simulink model "svpwm"  (R2024b)
settings: Solver=FixedStepAuto  StartTime=0.0  StopTime=0.02  FixedStep=1e-6  RelTol=1e-3
libraries: spsIGBTDiodeLib x6, simulink x5, spsDCVoltageSourceLib x1, spsThreePhaseSeriesRLCLoadLib x1, spsThreePhaseVIMeasurementLib x1, sps_lib x1
settings Model: Creator=killa  LastModifiedBy=killa

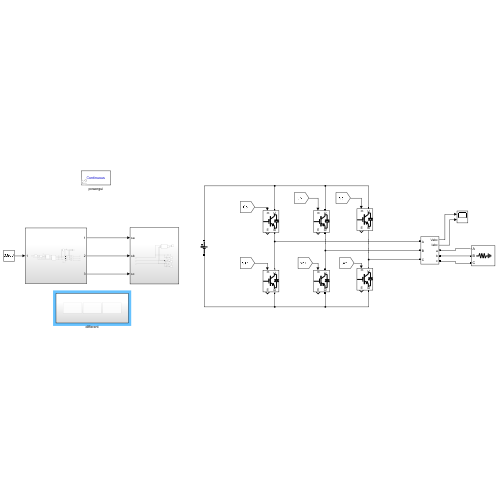
[thumbnail: Simulink's stored preview of the top-level diagram]
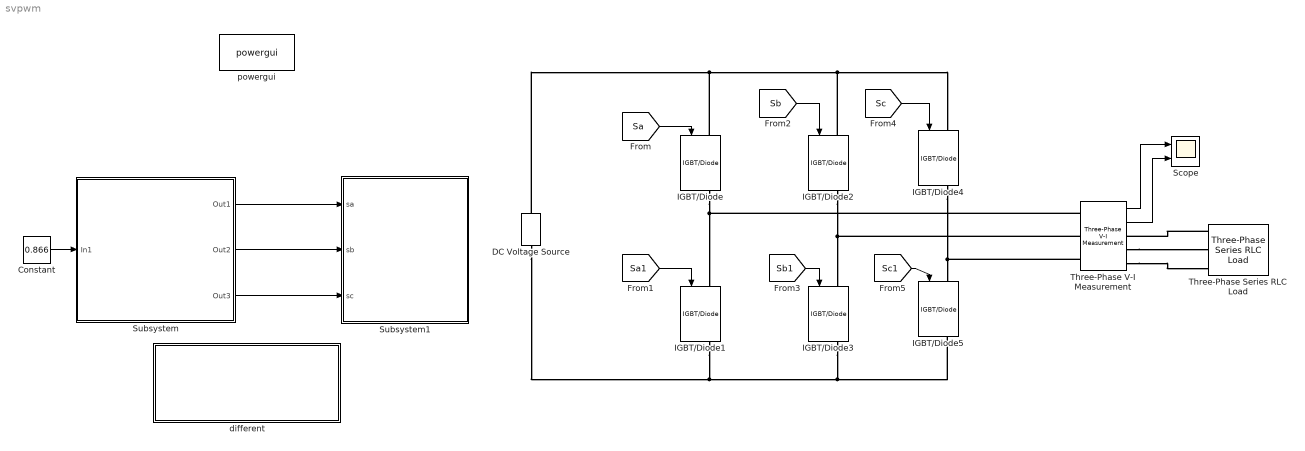
== system svpwm ==
  Constant : Constant  Value=0.866
  DC Voltage Source : spsDCVoltageSourceLib/DC Voltage Source  Amplitude=600  Measurements=None
  IGBT/Diode{,1..5} (6 alike) : spsIGBTDiodeLib/IGBT//Diode  Ron=1e-3  Rs=1e5  Cs=inf  Measurements=on
  Scope : Scope  NumInputPorts=2
  Subsystem : Subsystem
  Subsystem1 : Subsystem
  Three-Phase Series RLC Load : spsThreePhaseSeriesRLCLoadLib/Three-Phase Series RLC Load  LConnTagsString=A|B|C  Configuration=Y (grounded)  NominalVoltage=415  Vabc=[1e3 1e3 1e3]  Vabcp=[1e3 1e3 1e3]  NominalFrequency=50  UnbalancedPower=off  ActivePower=10e3  InductivePower=0  CapacitivePower=0  Pabc=[10e3 9e3 11e3]  QLabc=[100 90 110]  QCabc=[100 90 110]  Pabcp=[10e3 9e3 11e3]  QLabcp=[100 90 110]  QCabcp=[100 90 110]  Measurements=Branch currents  LoadType=constant Z
  Three-Phase V-I Measurement : spsThreePhaseVIMeasurementLib/Three-Phase V-I Measurement  VoltageMeasurement=phase-to-ground  SetLabelV=off  LabelV=Vabc  Vpu=off  VpuLL=off  CurrentMeasurement=yes  SetLabelI=off  LabelI=Iabc  Ipu=off  Pbase=100e6  Vbase=500e3  OutputType=Complex  PhasorSimulation=off  PSBequivalent=0
  different : Subsystem
  powergui : sps_lib/powergui  Priority=1  SimulationMode=Continuous  SampleTime=1e-6  frequency=60  Iterations=50  frequencyindice=0  Pbase=100e6  ErrMax=1e-4  UnitsV=kV  UnitsW=MW  buscounter=0  FunctionMessages=off  echomessages=off  EnableUseOfTLC=off  CurrentSourceSwitches=off  DisableSnubberDevices=off  DisableRonSwitches=off  DisableVfSwitches=off  DisplayEquations=off  AutomaticDiscreteSolvers=off  SolverType=Tustin/Backward Euler (TBE)  Interpol=off  ExternalGateDelay=off  methode=off  Ts=100  x0status=blocks  SPID=on  SwTol=0  HookPort=off  NonlinearTolerance=1e-4  nMaxIteration=100  ContinueOnMaxIteration=off  RestoreLinks=warning  ResistiveCurrentMeasurement=off  Frange=[0:2:500]  Ylog=off  Xlog=on  ShowGrid=off  save=off  variable=ZData  structure=0  ZoomFFT=off  StartTime=0.0  cycles=1  DisplayStyle=1  fundamental=60  FreqAxis=off  MaxFrequency=1000  frequencyindicesteady=1  RmsSteady=1  display=off
  wires:
  [Sa1] -> IGBT/Diode1/1
  [Sa] -> IGBT/Diode/1
  [Sb] -> IGBT/Diode2/1
  [Sb1] -> IGBT/Diode3/1
  [Sc] -> IGBT/Diode4/1
  [Sc1] -> IGBT/Diode5/1
  Three-Phase V-I Measurement/1 -> Scope/1
  Three-Phase V-I Measurement/2 -> Scope/2
  Constant/1 -> Subsystem/1(In1)
  Subsystem/1(Out1) -> Subsystem1/1(sa)
  Subsystem/2(Out2) -> Subsystem1/2(sb)
  Subsystem/3(Out3) -> Subsystem1/3(sc)
  connections:
  IGBT/Diode/LConn1 -- DC Voltage Source/RConn1 -- IGBT/Diode4/LConn1 -- IGBT/Diode2/LConn1
  IGBT/Diode/RConn1 -- Three-Phase V-I Measurement/LConn1 -- IGBT/Diode1/LConn1
  IGBT/Diode2/RConn1 -- Three-Phase V-I Measurement/LConn2 -- IGBT/Diode3/LConn1
  IGBT/Diode4/RConn1 -- Three-Phase V-I Measurement/LConn3 -- IGBT/Diode5/LConn1
  IGBT/Diode1/RConn1 -- DC Voltage Source/LConn1 -- IGBT/Diode3/RConn1 -- IGBT/Diode5/RConn1
  Three-Phase Series RLC Load/LConn1 -- Three-Phase V-I Measurement/RConn1
  Three-Phase V-I Measurement/RConn2 -- Three-Phase Series RLC Load/LConn2
  Three-Phase V-I Measurement/RConn3 -- Three-Phase Series RLC Load/LConn3

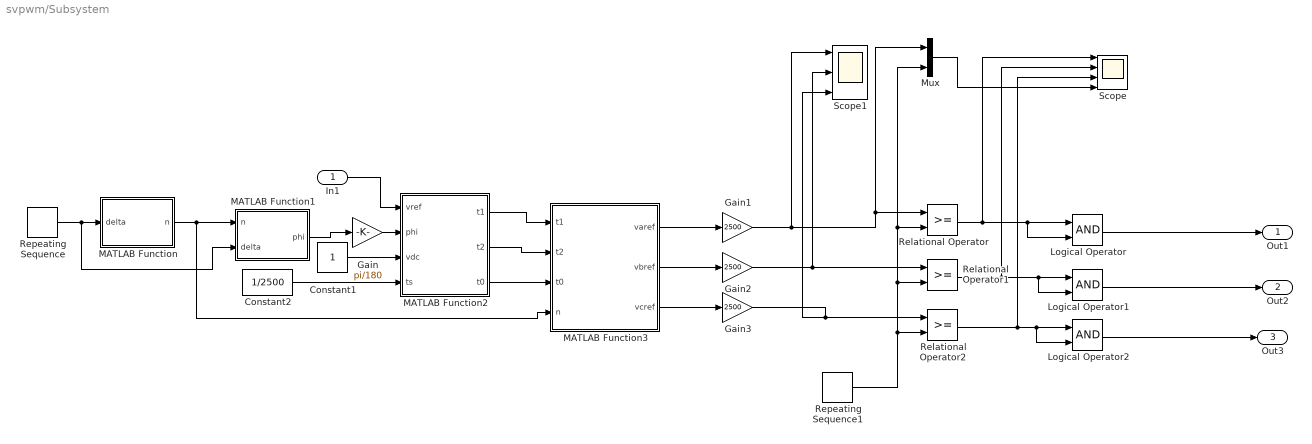
== system svpwm/Subsystem ==
  In1 : Inport
  Constant1 : Constant
  Constant2 : Constant  Value=1/2500
  Gain : Gain  Gain=pi/180
  Gain1 : Gain  Gain=2500
  Gain2 : Gain  Gain=2500
  Gain3 : Gain  Gain=2500
  Logical Operator : Logic  AllPortsSameDT=off  OutDataTypeStr=boolean
  Logical Operator1 : Logic  AllPortsSameDT=off  OutDataTypeStr=boolean
  Logical Operator2 : Logic  AllPortsSameDT=off  OutDataTypeStr=boolean
  MATLAB Function : MATLAB Function  TreatAsAtomicUnit=on
  MATLAB Function1 : MATLAB Function  TreatAsAtomicUnit=on
  MATLAB Function2 : MATLAB Function  TreatAsAtomicUnit=on
  MATLAB Function3 : MATLAB Function  TreatAsAtomicUnit=on
  Mux : Mux  Inputs=2
  Relational Operator : RelationalOperator  OutDataTypeStr=boolean  RndMeth=Simplest  InputSameDT=off
  Relational Operator1 : RelationalOperator  OutDataTypeStr=boolean  RndMeth=Simplest  InputSameDT=off
  Relational Operator2 : RelationalOperator  OutDataTypeStr=boolean  RndMeth=Simplest  InputSameDT=off
  Repeating Sequence : simulink/Sources/Repeating Sequence  rep_seq_t=[0 0.02]  rep_seq_y=[0 360]
  Repeating Sequence1 : simulink/Sources/Repeating Sequence  rep_seq_t=[0 0.5 1]/2500  rep_seq_y=[0 1 0]
  Scope : Scope  NumInputPorts=4
  Scope1 : Scope  NumInputPorts=3
  Out1 : Outport
  Out2 : Outport  Port=2
  Out3 : Outport  Port=3
  wires:
  Constant2/1 -> MATLAB Function2/4(ts)
  Repeating Sequence/1 -> MATLAB Function1/2(delta), MATLAB Function/1(delta)
  In1/1 -> MATLAB Function2/1(vref)
  Logical Operator/1 -> Out1/1
  MATLAB Function3/3(vcref) -> Gain3/1
  Logical Operator1/1 -> Out2/1
  Repeating Sequence1/1 -> Relational Operator2/2, Relational Operator1/2, Relational Operator/2, Mux/2
  MATLAB Function2/1(t1) -> MATLAB Function3/1(t1)
  Gain1/1 -> Scope1/1, Mux/1, Relational Operator/1
  Relational Operator/1 -> Scope/1, Logical Operator/2, Logical Operator/1
  Gain3/1 -> Relational Operator2/1, Scope1/3
  MATLAB Function2/3(t0) -> MATLAB Function3/3(t0)
  MATLAB Function3/1(varef) -> Gain1/1
  MATLAB Function2/2(t2) -> MATLAB Function3/2(t2)
  Relational Operator1/1 -> Scope/2, Logical Operator1/2, Logical Operator1/1
  Gain/1 -> MATLAB Function2/2(phi)
  MATLAB Function3/2(vbref) -> Gain2/1
  MATLAB Function1/1(phi) -> Gain/1
  MATLAB Function/1(n) -> MATLAB Function1/1(n), MATLAB Function3/4(n)
  Relational Operator2/1 -> Scope/3, Logical Operator2/2, Logical Operator2/1
  Gain2/1 -> Relational Operator1/1, Scope1/2
  Constant1/1 -> MATLAB Function2/3(vdc)
  Logical Operator2/1 -> Out3/1
  Mux/1 -> Scope/4

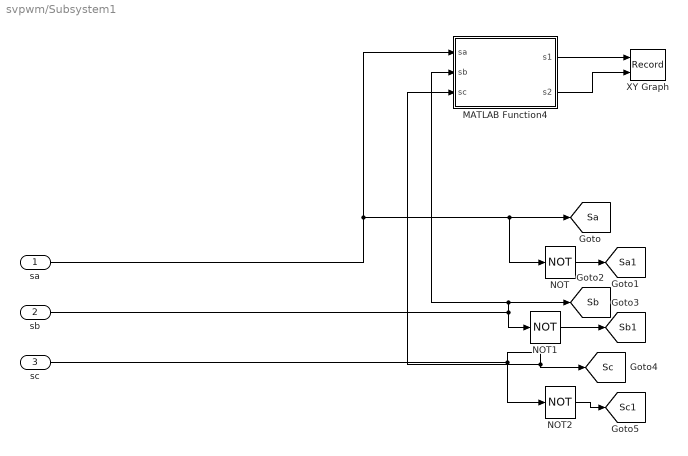
== system svpwm/Subsystem1 ==
  sa : Inport
  sb : Inport  Port=2
  sc : Inport  Port=3
  MATLAB Function4 : MATLAB Function  TreatAsAtomicUnit=on
  NOT : Logic  Operator=NOT  IconShape=distinctive  AllPortsSameDT=off  OutDataTypeStr=boolean
  NOT1 : Logic  Operator=NOT  IconShape=distinctive  AllPortsSameDT=off  OutDataTypeStr=boolean
  NOT2 : Logic  Operator=NOT  IconShape=distinctive  AllPortsSameDT=off  OutDataTypeStr=boolean
  XY Graph : Record  FileSettingsInternal="{\"entries\":[{\"content\":{\"excelSettings\":{\"content\":{},\"type\":\"Streamout.ExcelSettings\"}},\"type\":\"Streamout.FileSettingStorage\",\"uuid\":\"\"}],\"packageUris\":[\"http:\\/\\/schema.mathworks.com\\/mf0\\/streamout_blocks\\/R2020a\"],\"version\":\"1.0\"}"  Layout=[1 1]  SignalsInternal="{\"entries\":[{\"content\":{\"signals\":[{\"content\":{\"blockPath\":[],\"dimensions\":[1],\"domain\":\"\",\"lineColor\":\"#a2142f\",\"plots\":[ 1 ],\"port\":1,\"sid\":[\"\"],\"signalID\":1,\"signalName\":\"MATLAB Function4:1\"},\"type\":\"RecordBlkView.Signal\",\"uuid\":\"\"},{\"content\":{\"blockPath\":[],\"dimensions\":[1],\"domain\":\"\",\"lineColor\":\"#139fff\",\"plots\":[ 1 ],\"port\":2,\"sid\":[\"\"],\"signalID\":2,\"signalName\":\"MATLAB Function4:2\"},\"type\":\"RecordBlkView.Signal\",\"uuid\":\"\"}]},\"type\":\"RecordBlkView.InputSignals\",\"uuid\":\"\"}],\"packageUris\":[\"http:\\/\\/schema.mathworks.com\\/mf0\\/streamout_blocks\\/R2020a\"],\"version\":\"1.0\"}"  VisualizationBindings="{\"xyplotplugin\":{\"info\":[{\"series\":[{\"bindingParametersList\":[{\"parameter\":\"X-Axis\",\"signalID\":1,\"signalName\":\"MATLAB Function4:1\"},{\"parameter\":\"Y-Axis\",\"signalID\":2,\"signalName\":\"MATLAB Function4:2\"}],\"seriesID\":0}],\"subplotID\":1}]}}"  CompatibilityTag=XY
  tag scope: Sa1=global, Sa=global, Sb1=global, Sb=global, Sc1=global, Sc=global
  wires:
  MATLAB Function4/2(s2) -> XY Graph/2
  sa/1 -> MATLAB Function4/1(sa), NOT/1, [Sa]
  MATLAB Function4/1(s1) -> XY Graph/1
  sc/1 -> MATLAB Function4/3(sc), [Sc], NOT2/1
  sb/1 -> [Sb], MATLAB Function4/2(sb), NOT1/1
  NOT1/1 -> [Sb1]
  NOT2/1 -> [Sc1]
  NOT/1 -> [Sa1]

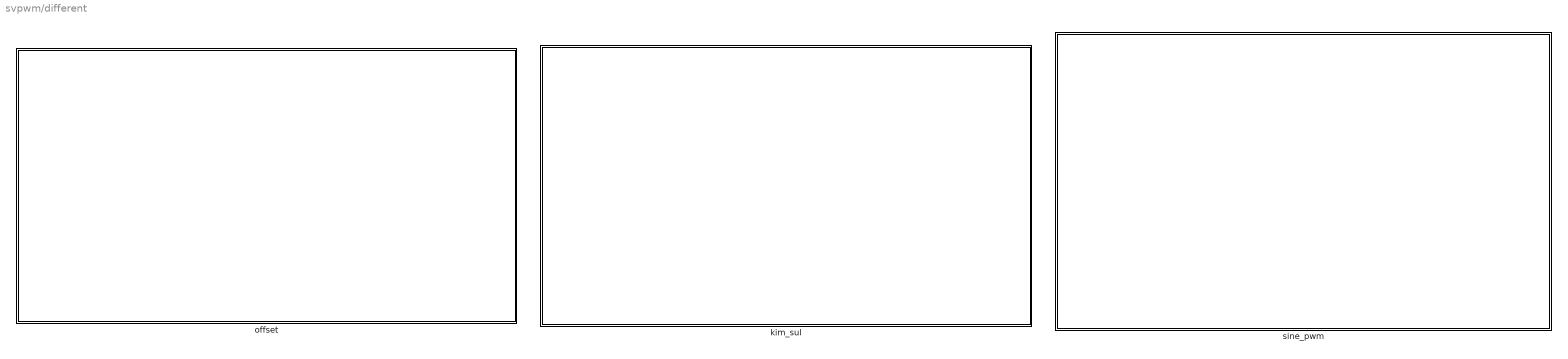
== system svpwm/different ==
  kim_sul : Subsystem
  offset : Subsystem
  sine_pwm : Subsystem

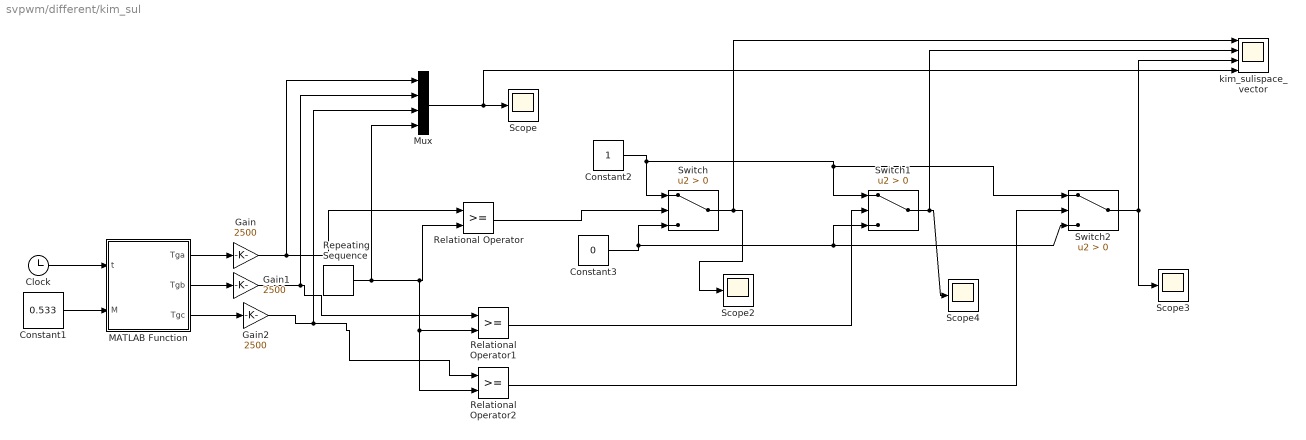
== system svpwm/different/kim_sul ==
  Clock : Clock
  Constant1 : Constant  Value=0.533
  Constant2 : Constant
  Constant3 : Constant  Value=0
  Gain : Gain  Gain=2500
  Gain1 : Gain  Gain=2500
  Gain2 : Gain  Gain=2500
  MATLAB Function : MATLAB Function  TreatAsAtomicUnit=on
  Mux : Mux
  Relational Operator : RelationalOperator  OutDataTypeStr=boolean  RndMeth=Simplest  InputSameDT=off
  Relational Operator1 : RelationalOperator  OutDataTypeStr=boolean  RndMeth=Simplest  InputSameDT=off
  Relational Operator2 : RelationalOperator  OutDataTypeStr=boolean  RndMeth=Simplest  InputSameDT=off
  Repeating Sequence : simulink/Sources/Repeating Sequence  rep_seq_t=[0 0.5 1]/2500  rep_seq_y=[0 1 0]
  Scope{,2..4} (4 alike) : Scope
  Switch : Switch  Criteria=u2 > Threshold  SaturateOnIntegerOverflow=off  InputSameDT=off
  Switch1 : Switch  Criteria=u2 > Threshold  SaturateOnIntegerOverflow=off  InputSameDT=off
  Switch2 : Switch  Criteria=u2 > Threshold  SaturateOnIntegerOverflow=off  InputSameDT=off
  kim_sulispace_vector : Scope  NumInputPorts=4
  wires:
  Repeating Sequence/1 -> Mux/4, Relational Operator2/2, Relational Operator1/2, Relational Operator/2
  MATLAB Function/1(Tga) -> Gain/1
  MATLAB Function/2(Tgb) -> Gain1/1
  MATLAB Function/3(Tgc) -> Gain2/1
  Constant1/1 -> MATLAB Function/2(M)
  Clock/1 -> MATLAB Function/1(t)
  Gain/1 -> Mux/1, Relational Operator/1
  Gain1/1 -> Mux/2, Relational Operator1/1
  Gain2/1 -> Mux/3, Relational Operator2/1
  Relational Operator2/1 -> Switch2/2
  Switch/1 -> kim_sulispace_vector/1, Scope2/1
  Constant3/1 -> Switch2/3, Switch1/3, Switch/3
  Constant2/1 -> Switch2/1, Switch1/1, Switch/1
  Relational Operator1/1 -> Switch1/2
  Switch1/1 -> kim_sulispace_vector/2, Scope4/1
  Relational Operator/1 -> Switch/2
  Switch2/1 -> kim_sulispace_vector/3, Scope3/1
  Mux/1 -> kim_sulispace_vector/4, Scope/1

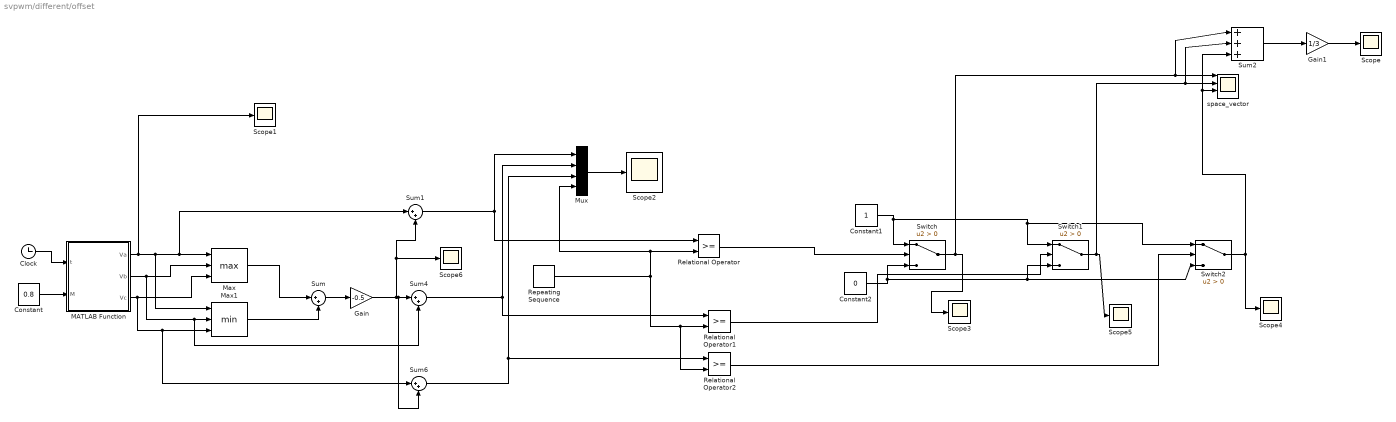
== system svpwm/different/offset ==
  Clock : Clock
  Constant : Constant  Value=0.8
  Constant1 : Constant
  Constant2 : Constant  Value=0
  Gain : Gain  Gain=-0.5
  Gain1 : Gain  Gain=1/3
  MATLAB Function : MATLAB Function  TreatAsAtomicUnit=on
  Max : MinMax  Function=max  Inputs=3
  Max1 : MinMax  Inputs=3
  Mux : Mux
  Relational Operator : RelationalOperator  OutDataTypeStr=boolean  RndMeth=Simplest  InputSameDT=off
  Relational Operator1 : RelationalOperator  OutDataTypeStr=boolean  RndMeth=Simplest  InputSameDT=off
  Relational Operator2 : RelationalOperator  OutDataTypeStr=boolean  RndMeth=Simplest  InputSameDT=off
  Repeating Sequence : simulink/Sources/Repeating Sequence  rep_seq_t=[0 0.5 1]/2500  rep_seq_y=[-1 1 -1]
  Scope{,1..6} (7 alike) : Scope
  Sum{,1,4,6} (4 alike) : Sum  Inputs=|++
  Sum2 : Sum  Inputs=|+++
  Switch : Switch  Criteria=u2 > Threshold  SaturateOnIntegerOverflow=off  InputSameDT=off
  Switch1 : Switch  Criteria=u2 > Threshold  SaturateOnIntegerOverflow=off  InputSameDT=off
  Switch2 : Switch  Criteria=u2 > Threshold  SaturateOnIntegerOverflow=off  InputSameDT=off
  space_vector : Scope  NumInputPorts=4
  wires:
  Sum/1 -> Gain/1
  Max/1 -> Sum/1
  Gain/1 -> Sum1/2, Scope6/1, Sum6/2, Sum4/1
  Max1/1 -> Sum/2
  Repeating Sequence/1 -> Relational Operator/2, Mux/4, Relational Operator2/2, Relational Operator1/2
  Clock/1 -> MATLAB Function/1(t)
  Sum1/1 -> Mux/1, Relational Operator/1
  Sum4/1 -> Mux/2, Relational Operator1/1
  Sum6/1 -> Mux/3, Relational Operator2/1
  Constant/1 -> MATLAB Function/2(M)
  MATLAB Function/1(Va) -> Scope1/1, Max1/1, Sum1/1, Max/1
  MATLAB Function/2(Vb) -> Sum4/2, Max1/2, Max/2
  MATLAB Function/3(Vc) -> Sum6/1, Max1/3, Max/3
  Switch1/1 -> Sum2/2, space_vector/2, Scope5/1
  Switch2/1 -> Sum2/3, space_vector/3, Scope4/1
  Switch/1 -> Sum2/1, space_vector/1, Scope3/1
  Constant2/1 -> Switch2/3, Switch1/3, Switch/3
  Relational Operator1/1 -> Switch1/2
  Constant1/1 -> Switch2/1, Switch1/1, Switch/1
  Relational Operator/1 -> Switch/2
  Relational Operator2/1 -> Switch2/2
  Sum2/1 -> Gain1/1
  Gain1/1 -> Scope/1
  Mux/1 -> Scope2/1

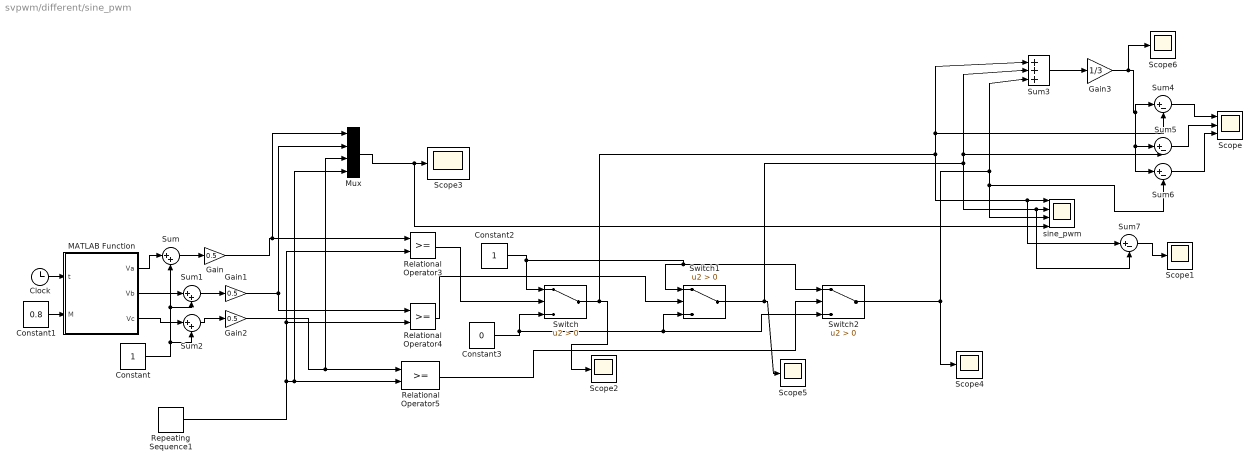
== system svpwm/different/sine_pwm ==
  Clock : Clock
  Constant : Constant
  Constant1 : Constant  Value=0.8
  Constant2 : Constant
  Constant3 : Constant  Value=0
  Gain : Gain  Gain=0.5
  Gain1 : Gain  Gain=0.5
  Gain2 : Gain  Gain=0.5
  Gain3 : Gain  Gain=1/3
  MATLAB Function : MATLAB Function  TreatAsAtomicUnit=on
  Mux : Mux
  Relational Operator3 : RelationalOperator  OutDataTypeStr=boolean  RndMeth=Simplest  InputSameDT=off
  Relational Operator4 : RelationalOperator  OutDataTypeStr=boolean  RndMeth=Simplest  InputSameDT=off
  Relational Operator5 : RelationalOperator  OutDataTypeStr=boolean  RndMeth=Simplest  InputSameDT=off
  Repeating Sequence1 : simulink/Sources/Repeating Sequence  rep_seq_t=[0 0.5 1]/2500  rep_seq_y=[0 1 0]
  Scope : Scope  NumInputPorts=3
  Scope{1..6} (6 alike) : Scope
  Sum : Sum  Inputs=|++
  Sum1 : Sum  Inputs=|++
  Sum2 : Sum  Inputs=|++
  Sum3 : Sum  Inputs=|+++
  Sum{4..7} (4 alike) : Sum  Inputs=|+-
  Switch : Switch  Criteria=u2 > Threshold  SaturateOnIntegerOverflow=off  InputSameDT=off
  Switch1 : Switch  Criteria=u2 > Threshold  SaturateOnIntegerOverflow=off  InputSameDT=off
  Switch2 : Switch  Criteria=u2 > Threshold  SaturateOnIntegerOverflow=off  InputSameDT=off
  sine_pwm : Scope  NumInputPorts=4
  wires:
  Repeating Sequence1/1 -> Relational Operator4/2, Relational Operator3/2, Mux/4, Relational Operator5/2
  Sum/1 -> Gain/1
  Sum1/1 -> Gain1/1
  Sum2/1 -> Gain2/1
  Constant/1 -> Sum2/2, Sum1/2, Sum/2
  Gain/1 -> Mux/1, Relational Operator3/1
  Gain1/1 -> Mux/2, Relational Operator4/1
  MATLAB Function/1(Va) -> Sum/1
  MATLAB Function/2(Vb) -> Sum1/1
  MATLAB Function/3(Vc) -> Sum2/1
  Clock/1 -> MATLAB Function/1(t)
  Constant1/1 -> MATLAB Function/2(M)
  Relational Operator4/1 -> Switch1/2
  Relational Operator3/1 -> Switch/2
  Relational Operator5/1 -> Switch2/2
  Sum6/1 -> Scope/3
  Switch1/1 -> Sum5/2, Sum3/2, Sum7/2, sine_pwm/2, Scope5/1
  Constant3/1 -> Switch2/3, Switch1/3, Switch/3
  Constant2/1 -> Switch2/1, Switch1/1, Switch/1
  Sum4/1 -> Scope/1
  Sum7/1 -> Scope1/1
  Switch2/1 -> Sum3/3, Sum6/2, sine_pwm/3, Scope4/1
  Gain3/1 -> Scope6/1, Sum6/1, Sum5/1, Sum4/1
  Sum3/1 -> Gain3/1
  Sum5/1 -> Scope/2
  Switch/1 -> Sum4/2, Sum3/1, Sum7/1, sine_pwm/1, Scope2/1
  Mux/1 -> sine_pwm/4, Scope3/1
  Gain2/1 -> Mux/3, Relational Operator5/1

== matlab function svpwm/Subsystem/MATLAB Function1 ==
  data: n input; delta input; phi output
function phi = phi(n,delta)
phi=0;
if n==1 
    phi=delta;
end
if n==2 
    phi=delta-60;
end
if n==3 
    phi=delta-120;
end
if n==4 
    phi=delta-180;
end
if n==5 
    phi=delta-240;
end
if n==6 
    phi=delta-300;
end

end

== matlab function svpwm/Subsystem/MATLAB Function ==
  data: delta input; n output
function n = sector(delta)
n=0;
if delta>=0 && delta<=60
    n=1;
end
if delta>=60 && delta<=120
    n=2;
end
if delta>=120 && delta<=180
    n=3;
end
if delta>=180 && delta<=240
    n=4;
end
if delta>=240 && delta<=300
    n=5;
end
if delta>=300 && delta<=360
    n=6;
end
end

== matlab function svpwm/Subsystem/MATLAB Function2 ==
  data: vref input; phi input; t1 output; vdc input; ts input; t2 output; t0 output
function [t1,t2,t0] = timings(vref,phi,vdc,ts)
t1=ts*(vref/vdc)*sin((pi/3)-phi)/sin(pi/3);
t2=ts*(vref/vdc)*sin(phi)/sin(pi/3);
t0=ts-(t1+t2);
end

== matlab function svpwm/Subsystem/MATLAB Function3 ==
  data: t1 input; t2 input; t0 input; n input; varef output; vbref output; vcref output
function [varef,vbref,vcref] = vref(t1,t2,t0,n)
varef=0;vbref=0;vcref=0;
if n==1
    varef=t1+t2+t0/2;
    vbref=t2+t0/2;
    vcref=t0/2;
end
if n==2
    varef=t1+t0/2;
    vbref=t1+t2+t0/2;
    vcref=t0/2;
end
if n==3
    varef=t0/2;
    vbref=t1+t2+t0/2;
    vcref=t2+t0/2;
end
if n==4
    varef=t0/2;
    vbref=t1+t0/2;
    vcref=t1+t2+t0/2;
end
if n==5
    varef=t2+t0/2;
    vbref=t0/2;
    vcref=t1+t2+t0/2;
end
if n==6
    varef=t1+t2+t0/2;
    vbref=t0/2;
    vcref=t1+t0/2;
end
end

== matlab function svpwm/Subsystem1/MATLAB Function4 ==
  data: sa input; s1 output; sb input; sc input; s2 output
function [s1,s2] = space_vector(sa,sb,sc)
s1=sa*cos(0)+sb*cos(2*pi/3)+sc*cos(4*pi/3);
s2=sa*sin(0)+sb*sin(2*pi/3)+sc*sin(4*pi/3);
end

== matlab function svpwm/different/kim_sul/MATLAB Function ==
  data: t input; Tga output; M input; Tgb output; Tgc output
function [Tga,Tgb,Tgc] = ...
          KimSulSVPWM(t,M)
% Parameters
f = 50;          % Fundamental frequency (Hz)         % Modulation index (Amplitude)

% Angular frequency
w = 2*pi*f;

% Three-phase sine waves
Va = M*sin(w*t);
Vb = M*sin(w*t - 2*pi/3);   % -120 degrees
Vc = M*sin(w*t + 2*pi/3);   % +120 degrees
%#codegen

%% Equivalent Time Signals
Ts=(1/2500);
Vdc= 1;
Ta = Ts*Va/Vdc;
Tb = Ts*Vb/Vdc;
Tc = Ts*Vc/Vdc;

%% Maximum

Tmax = max([Ta Tb Tc]);

%% Minimum

Tmin = min([Ta Tb Tc]);

%% Effective Vector Time

Teff = Tmax - Tmin;

%% Zero Vector Time

Tzero = Ts - Teff;

%% Offset Time

Toffset = Tzero/2 - Tmin;

%% Final Switching Times

Tga = Ta + Toffset;
Tgb = Tb + Toffset;
Tgc = Tc + Toffset;

end

== matlab function svpwm/different/sine_pwm/MATLAB Function ==
  data: t input; Va output; Vb output; Vc output; M input
function [Va, Vb, Vc] = fcn(t,M)

% Parameters
f = 50;          % Fundamental frequency (Hz)         % Modulation index (Amplitude)

% Angular frequency
w = 2*pi*f;

% Three-phase sine waves
Va = M*sin(w*t);
Vb = M*sin(w*t - 2*pi/3);   % -120 degrees
Vc = M*sin(w*t + 2*pi/3);   % +120 degrees

end

== matlab function svpwm/different/offset/MATLAB Function ==
  data: t input; Va output; Vb output; Vc output; M input
function [Va, Vb, Vc] = fcn(t, M)

% Parameters
f = 50;              % Fundamental frequency (Hz)

% Angular frequency
w = 2*pi*f;

% Three-phase pure sine waves
Va = M * sin(w*t);
Vb = M * sin(w*t - 2*pi/3);   % -120°
Vc = M * sin(w*t + 2*pi/3);   % +120°

end
